simulink model "sla_quadratic_formula"  (R2015b)
settings: Solver=FixedStepDiscrete  SolverMode=SingleTasking  StartTime=0.0  StopTime=10.0  RelTol=1e-3
settings Model: DataTypeOverride=Off  Creator=amatsumo  LastModifiedBy=amatsumo
settings DataIOCC: SaveFormat=Array  SaveOutput=off  SaveTime=off
settings OptimizationCC: BlockReduction=off  ConditionallyExecuteInputs=off  DefaultParameterBehavior=Inlined
settings DebuggingCC: AlgebraicLoopMsg=error  SolverPrmCheckMsg=warning  SingleTaskRateTransMsg=error
settings HardwareCC: ProdBitPerPointer=32  ProdLargestAtomicFloat=None  ProdIntDivRoundTo=Undefined  ProdEndianess=Unspecified  ProdWordSize=32  ProdHWDeviceType=ASIC/FPGA->ASIC/FPGA  ProdEqTarget=off
settings GRTTargetCC: GeneratePreprocessorConditionals=Disable all
settings ConfigComp: CovModelRefEnable=Off  CovSFcnEnable=off

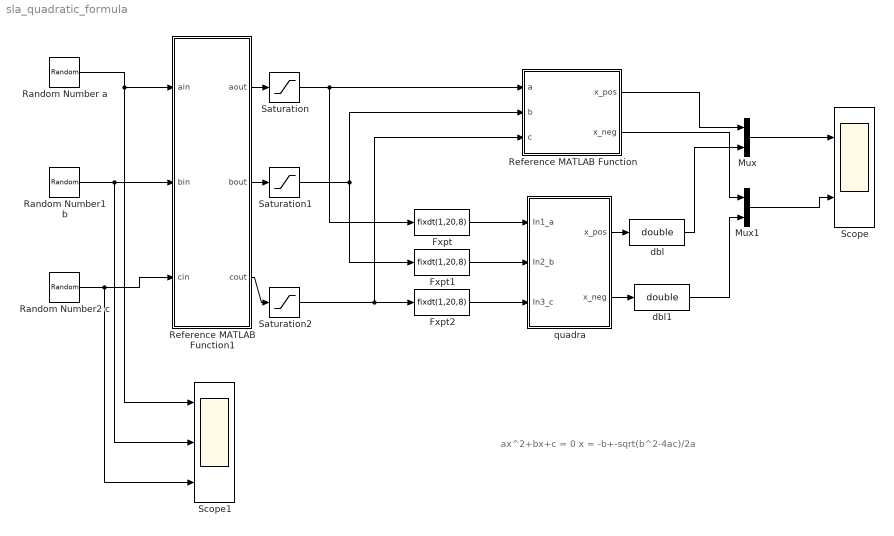
== system sla_quadratic_formula ==
  note: ax^2+bx+c = 0
      | x = -b+-sqrt(b^2-4ac)/2a
  Fxpt : DataTypeConversion  OutDataTypeStr=fixdt(1,20,8)
  Fxpt1 : DataTypeConversion  OutDataTypeStr=fixdt(1,20,8)
  Fxpt2 : DataTypeConversion  OutDataTypeStr=fixdt(1,20,8)
  Mux : Mux  Inputs=2
  Mux1 : Mux  Inputs=2
  Random Number a : RandomNumber  Variance=8  Seed=1  SampleTime=1
  Random Number1 b : RandomNumber  Variance=8  Seed=2  SampleTime=1
  Random Number2 c : RandomNumber  Variance=8  Seed=3  SampleTime=1
  Reference MATLAB Function : MATLAB Function  TreatAsAtomicUnit=on
  Reference MATLAB Function1 : MATLAB Function  TreatAsAtomicUnit=on
  Saturation : Saturate  UpperLimit=7.99  LowerLimit=-8
  Saturation1 : Saturate  UpperLimit=7.99  LowerLimit=-8
  Saturation2 : Saturate  UpperLimit=7.99  LowerLimit=-8
  Scope : Scope  NumInputPorts=2
  Scope1 : Scope  NumInputPorts=3
  dbl : DataTypeConversion  OutDataTypeStr=double
  dbl1 : DataTypeConversion  OutDataTypeStr=double
  quadra : Subsystem
  wires:
  Reference MATLAB Function1/1(aout) -> Saturation/1
  Reference MATLAB Function1/2(bout) -> Saturation1/1
  Reference MATLAB Function1/3(cout) -> Saturation2/1
  Reference MATLAB Function/1(x_pos) -> Mux/1
  quadra/1(x_pos) -> dbl/1
  Reference MATLAB Function/2(x_neg) -> Mux1/1
  quadra/2(x_neg) -> dbl1/1
  Mux/1 -> Scope/1
  Mux1/1 -> Scope/2
  Random Number a/1 -> Scope1/1, Reference MATLAB Function1/1(ain)
  Random Number1 b/1 -> Scope1/2, Reference MATLAB Function1/2(bin)
  Random Number2 c/1 -> Scope1/3, Reference MATLAB Function1/3(cin)
  Saturation/1 -> Fxpt/1, Reference MATLAB Function/1(a)
  Saturation1/1 -> Fxpt1/1, Reference MATLAB Function/2(b)
  Saturation2/1 -> Fxpt2/1, Reference MATLAB Function/3(c)
  Fxpt/1 -> quadra/1(In1_a)
  Fxpt1/1 -> quadra/2(In2_b)
  Fxpt2/1 -> quadra/3(In3_c)
  dbl/1 -> Mux/2
  dbl1/1 -> Mux1/2

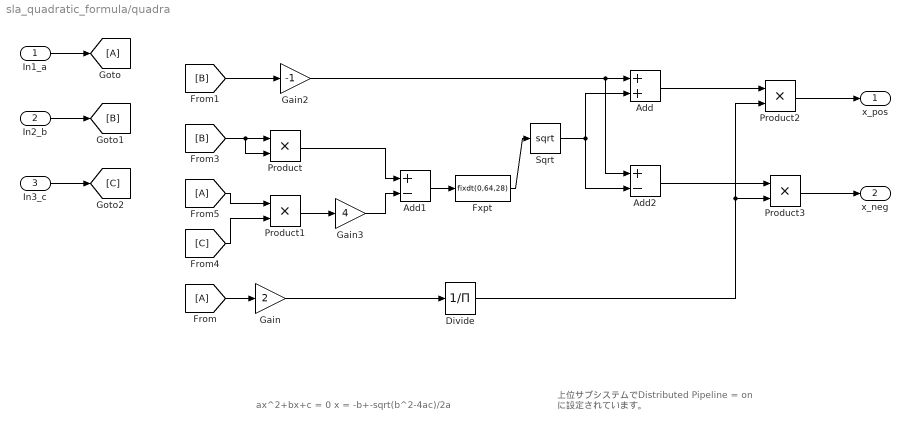
== system sla_quadratic_formula/quadra ==
  note: 上位サブシステムでDistributed Pipeline = on
      | に設定されています。
  note: ax^2+bx+c = 0
      | x = -b+-sqrt(b^2-4ac)/2a
  In1_a : Inport
  In2_b : Inport  Port=2
  In3_c : Inport  Port=3
  Add : Sum
  Add1 : Sum  Inputs=+-
  Add2 : Sum  Inputs=+-
  Divide : Product  Inputs=/  SaturateOnIntegerOverflow=on  RndMeth=Zero
  Fxpt : DataTypeConversion  OutDataTypeStr=fixdt(0,64,28)  SaturateOnIntegerOverflow=on
  Gain : Gain  Gain=2  OutDataTypeStr=Inherit: Same as input
  Gain2 : Gain  Gain=-1  OutDataTypeStr=Inherit: Same as input
  Gain3 : Gain  Gain=4  OutDataTypeStr=Inherit: Same as input
  Product : Product
  Product1 : Product
  Product2 : Product  RndMeth=Zero
  Product3 : Product  RndMeth=Zero
  Sqrt : Sqrt  SaturateOnIntegerOverflow=on
  x_pos : Outport
  x_neg : Outport  Port=2
  wires:
  Fxpt/1 -> Sqrt/1
  Add2/1 -> Product3/1
  Product3/1 -> x_neg/1
  Product2/1 -> x_pos/1
  Divide/1 -> Product3/2, Product2/2
  Gain/1 -> Divide/1
  [A] -> Gain/1
  Add/1 -> Product2/1
  Add1/1 -> Fxpt/1
  Gain3/1 -> Add1/2
  Product/1 -> Add1/1
  Product1/1 -> Gain3/1
  [C] -> Product1/2
  [A] -> Product1/1
  [B] -> Product/2, Product/1
  Sqrt/1 -> Add2/2, Add/2
  Gain2/1 -> Add2/1, Add/1
  [B] -> Gain2/1
  In3_c/1 -> [C]
  In2_b/1 -> [B]
  In1_a/1 -> [A]

== matlab function sla_quadratic_formula/Reference MATLAB Function1 ==
  data: ain input; aout output; bin input; cin input; bout output; cout output
function [aout,bout,cout] = fcn(ain,bin,cin)
%#eml

% sqrtが複素数にならないよう入力値の制限

if (bin^2-4*ain*cin)>=0
	aout = ain;
	bout = bin;
	cout = cin;
else
	aout = -ain;
	bout = bin;
	cout = cin;
end

== matlab function sla_quadratic_formula/Reference MATLAB Function ==
  data: a input; x_pos output; b input; c input; x_neg output
function [x_pos,x_neg] = fcn(a,b,c)
%#eml

x_pos = (-b+sqrt(b^2-4*a*c))/(2*a);
x_neg = (-b-sqrt(b^2-4*a*c))/(2*a);
